simulink model "model_base_2fm"  (R2016b)
settings: Solver=FixedStepDiscrete  StartTime=0.0  StopTime=inf  FixedStep=sampleTime  RelTol=1e-3
PostLoadFcn:
  | % load model parameters
  | base_1fm_parameters;
  | 
  | % set requested state
  | set_param('model_base_2fm/Requested state','Value',num2str(0));
InitFcn:
  | % load model parameters
  | base_1fm_parameters;
  | 
  | % set requested state
  | set_param('model_base_2fm/Requested state','Value',num2str(0));
StartFcn:
  | % load model parameters
  | base_1fm_parameters;
  | 
  | % set requested state
  | set_param('model_base_2fm/Requested state','Value',num2str(0));
undefined symbols (not defined in the file or in its folder): FM1, Lb, Lf, Lu, sampleTime
undefined symbols (not defined in the file): FM2
libraries: simulink x21, LibraryFM x16, VariousBlocksLibrary x4, FMLibrary_v2 x1
(part 3 of 3)

== matlab function model_base_2fm/Robot2/DataFromEtherCAT/Calculate Arrange Joint and Op Space/forward kinematics1/Je ==
  data: q input; Je output size=[2 2]; Lf parameter; Lu parameter; Lb parameter
function Je = Je( q, Lf, Lu, Lb)
%#codegen

% Calculate the Jacobian for this particular device configuration.
% Note that the function func_eq_Je needs to be in the libraries/kinematis_functions folder

% jacobians
Je = func_eq_Je(q(1),q(2),Lf,Lu,Lb);

== matlab function model_base_2fm/Robot2/DataFromEtherCAT/Calculate Arrange Joint and Op Space/forward kinematics1/Jedot ==
  data: q input; qdot input; Jedot output size=[2 2]; Lf parameter; Lu parameter; Lb parameter
function Jedot = Jedot( q, qdot, Lf, Lu, Lb)
%#codegen

% Calculate the time derivative of the Jacobian for this particular device configuration.
% Note that the function func_eq_Je needs to be in the libraries/kinematis_functions folder


% jacobians
Jedot = func_eq_Jedot(q(1),q(2),qdot(1),qdot(2),Lf,Lu,Lb);

== matlab function model_base_2fm/Robot2/DataFromEtherCAT/Calculate Arrange Joint and Op Space/forward kinematics1/calculate xddot ==
  data: qddot input; qdot input size=[2 1]; J input; xddot output size=[2 1]; Jdot input
function xddot = calc_xddot(qddot, qdot, J, Jdot)
%#codegen

xddot = J*qddot + Jdot*qdot;

== matlab function model_base_2fm/Robot2/DataFromEtherCAT/Calculate Arrange Joint and Op Space/forward kinematics1/forward kinematics ==
  data: q input; x output size=[2 1]; Lf parameter; Lu parameter; Lb parameter
function x = FK(q, Lf, Lu, Lb)
%#codegen

% Calculate the endpoint position (forward kinematics)
% Note that the function func_eq_FK needs to be in the libraries/kinematis_functions folder


x = func_eq_FK(q(1),q(2),Lf,Lu,Lb);

== matlab function model_base_2fm/Robot2/DataFromEtherCAT/FTSensor_K6D27/CorrectOffset ==
  data: u_in input; u_out output; reset input; corrected output
function [u_out,corrected] = CorrectOffset(u_in,reset)
%#codegen

persistent data_ offset_ counter_ corrected_;
N = 1000;

% initialize
if isempty(data_)
    data_ = zeros(size(u_in,1), N);
    offset_ = zeros(size(u_in));
    counter_ = 1;
    corrected_ = 0;
end

if (counter_ <= N)
    data_(:,counter_) = u_in;
end

counter_ = counter_ + 1;
if reset
    counter_ = 1;
end

% calculate mean
if counter_ == N
    corrected_ = 1;
    offset_ = mean(data_,2);
end

corrected = corrected_;
u_out = u_in - offset_;

== matlab function model_base_2fm/Robot2/DataFromEtherCAT/FTSensor_K6D27/SensorToOperationalSpace ==
  data: q_all input; Fs input; FTOpSpace output; transmatside input
function FTOpSpace = ForceSensorToOperationalSpace(q_all,Fs,transmatside)
%#codegen
q1 = q_all(1);
q2 = q_all(2);
q4 = q_all(4);
q5 = q_all(5);

% based on which arm the force sensor is connected
switch transmatside
    case 1
        alpha = pi-q2;   
        beta = q1+alpha-pi/2;
        R0 = rotmat(beta);
        R = blkdiag(R0,R0); % transform forces and moments
    case 2
        alpha = -(pi - q4);
        beta = q5+alpha-pi/2;
        R0 = rotmat(beta);
        R = blkdiag(R0,R0); % transform forces and moments
    otherwise
        R = eye(length(Fs));
end

% transform force
FTOpSpace = R*Fs;

function R = rotmat(q)

R = [cos(q) -sin(q) 0;...
      sin(q)  cos(q) 0;...
      0       0      1];

== matlab function model_base_2fm/Robot2/DataToEtherCAT/FTSensorError/MATLAB Function ==
  data: ForcesTorques input; e output; MaxForcesTorques input
function e = fcn(ForcesTorques, MaxForcesTorques)

% throw error when any of the forces/torques go over a max allowable value
if any(abs(ForcesTorques) > MaxForcesTorques) 
    e = 1;
else
    e = 0;
end

== matlab function model_base_2fm/Robot2/DataToEtherCAT/WorkspacePositionGuard/CheckInternalAngles ==
  data: theta input; angleError output
function angleError = checkInternalErrors(theta)
%#codegen

angleError = 0;
if any(theta([2 4]) >= 0.95*pi)
    angleError = 1;
end

== matlab function model_base_2fm/Robot2/DataToEtherCAT/WorkspacePositionGuard/EndpointPositionGuard ==
  data: correctState input; xe input; error output
function error = fcn(correctState, xe)
%#codegen


error = 0;

% only check workspace boundaries after homing state is done
if ~correctState 
    return; 
end

% x0 = 0;
% y0 = 0.2354;
% a = 0.11;
% b = 0.08;

% workspace (see design document)
x0 = 0;
y0 = 0.25024;
a = 0.1746;
b = 0.13;%0.1048;

% check if endpoint is outside a predefined ellipse
x = xe(1);
y = xe(2);

% workspace is defined as an ellipse
e = (x-x0)^2 / a^2 + (y-y0)^2 / b^2;

% if is larger than 1, the endpoint is outside the workspace
if e > 1
    error = 1;
end

== matlab function model_base_2fm/Robot2/StateMachineLocal/CheckVelThreshold ==
  data: qdot input; velBelowThreshold output; threshold input
function velBelowThreshold = checkVelThreshold(qdot, threshold)

velBelowThreshold = all(abs(qdot) <= threshold);

== matlab function model_base_2fm/Robot2/StateMachineLocal/Encode system state change ==
  data: stateChanged input; state input; systemStateChanged output
function systemStateChanged  = fcn(stateChanged,state)

systemStateChanged = 0;


if stateChanged
    switch(state)
        case 201 % do calibration
            systemStateChanged = 1;
    end
end

== stateflow chart model_base_2fm/Robot2/StateMachineLocal/State machine ==
  state Idle
    en:
    currentState = 0;
  state Init
    en:
    currentState = 1;
    du:
    isInitialized = true;
  state Calibration
    en:
    currentState = 2;
    state JointVelLarge
    state JointVelSmall
    state DoCalibration
      en: currentState = 201;
    state CalibrationDone
      en: currentState = 299;
    (default) -> JointVelLarge
    JointVelSmall -> JointVelLarge [order 1] : [!velBelowThreshold]
    JointVelLarge -> JointVelSmall : [velBelowThreshold]
    JointVelSmall -> DoCalibration [order 2] : after(1,sec)
    DoCalibration -> CalibrationDone
  state Operational
    state Homing
      en:
      currentState = requestedState;
      state NotAtHome
      state AtHome
      state HomingDone
        en: currentState = 399;
      (default) -> NotAtHome
      AtHome -> NotAtHome [order 1] : [!isAtHome]
      NotAtHome -> AtHome : [isAtHome]
      AtHome -> HomingDone [order 2] : after(1,sec)
    state Run
      en: currentState = 4;
    Run -> Homing : [requestedState == 301 || requestedState == 302]
    HomingDone -> Run : [requestedState==4]
  state Error
    en: currentState=-1;
  (default) -> Idle
  Idle -> Init : [requestedState==1 || requestedState == 2]
  Init -> Calibration [order 2] : [requestedState==2]
  Init -> Idle [order 1] : [requestedState==0]
  Error -> Idle : [!fault && requestedState==0]
  Operational -> Idle [order 2] : [requestedState==0]
  CalibrationDone -> Homing : [requestedState == 301 || requestedState == 302]
  Operational -> Error [order 1] : [fault]
  data: requestedState input double; currentState output double; fault input boolean; isInitialized local double; velBelowThreshold input boolean; isAtHome input boolean

== matlab function model_base_2fm/Robot2/StateMachineLocal/checkEndpointPosition ==
  data: x input; homeLocation input; isAtEndpoint output; threshold input
function isAtEndpoint = checkEndpointPosition(x, homeLocation, threshold)
% check whether the endpoint position is within a specified circle with
% radius threshold and midopoint HomePosition

% calculate distance between home position and joint positions
d = sqrt(sum((homeLocation - x).^2));

if imag(d) || isinf(d) || isnan(d)
    isAtEndpoint = false;
else
    isAtEndpoint = (d <= threshold);
end

== matlab function model_base_2fm/Robot1/DataFromEtherCAT/FTSensor_K6D27/SensorToOperationalSpace ==
  data: q_all input; Fs input; FTOpSpace output; transmatside input
function FTOpSpace = ForceSensorToOperationalSpace(q_all,Fs,transmatside)
%#codegen
q1 = q_all(1);
q2 = q_all(2);
q4 = q_all(4);
q5 = q_all(5);

% based on which arm the force sensor is connected
switch transmatside
    case 1
        alpha = pi-q2;   
        beta = q1+alpha-pi/2;
        R0 = rotmat(beta);
        R = blkdiag(R0,R0); % transform forces and moments
    case 2
        alpha = -(pi - q4);
        beta = q5+alpha-pi/2;
        R0 = rotmat(beta);
        R = blkdiag(R0,R0); % transform forces and moments
    otherwise
        R = eye(length(Fs));
end

% transform force
FTOpSpace = R*Fs;

function R = rotmat(q)

R = [cos(q) -sin(q) 0;...
      sin(q)  cos(q) 0;...
      0       0      1];

== matlab function model_base_2fm/Robot1/DataToEtherCAT/WorkspacePositionGuard/CheckInternalAngles ==
  data: theta input; angleError output
function angleError = checkInternalErrors(theta)
%#codegen

angleError = 0;
if any(theta([2 4]) >= 0.95*pi)
    angleError = 1;
end

== matlab function model_base_2fm/Robot1/DataToEtherCAT/WorkspacePositionGuard/EndpointPositionGuard ==
  data: correctState input; xe input; error output
function error = fcn(correctState, xe)
%#codegen


error = 0;

% only check workspace boundaries after homing state is done
if ~correctState 
    return; 
end

% x0 = 0;
% y0 = 0.2354;
% a = 0.11;
% b = 0.08;

% workspace (see design document)
x0 = 0;
y0 = 0.25024;
a = 0.1746;
b = 0.13;%0.1048;

% check if endpoint is outside a predefined ellipse
x = xe(1);
y = xe(2);

% workspace is defined as an ellipse
e = (x-x0)^2 / a^2 + (y-y0)^2 / b^2;

% if is larger than 1, the endpoint is outside the workspace
if e > 1
    error = 1;
end
